simulink model "LdAfsSlave_Runner"  (R2020b)
settings: configuration reference "VLS_Standard_Configuration" (kept outside this file)
undefined symbols (not defined in the file): C_AfsRampTimeMatrix, C_CieCurveGammaToPwmY, C_CieCurvePwmToGammaY, C_DblSlavePeriod, C_EndIndexOfEachLightingModule, C_LedCenterDist, C_LedLeftDist, C_LedRightDist, C_StartIndexOfEachLightingModule
libraries: AfsSlaveLib x1
settings Model: DataDictionary=LdAfsDblSlaveDD.sldd  Creator=ahashem  LastModifiedBy=ahashem
settings ConfigSetRef: SourceName=VLS_Standard_Configuration

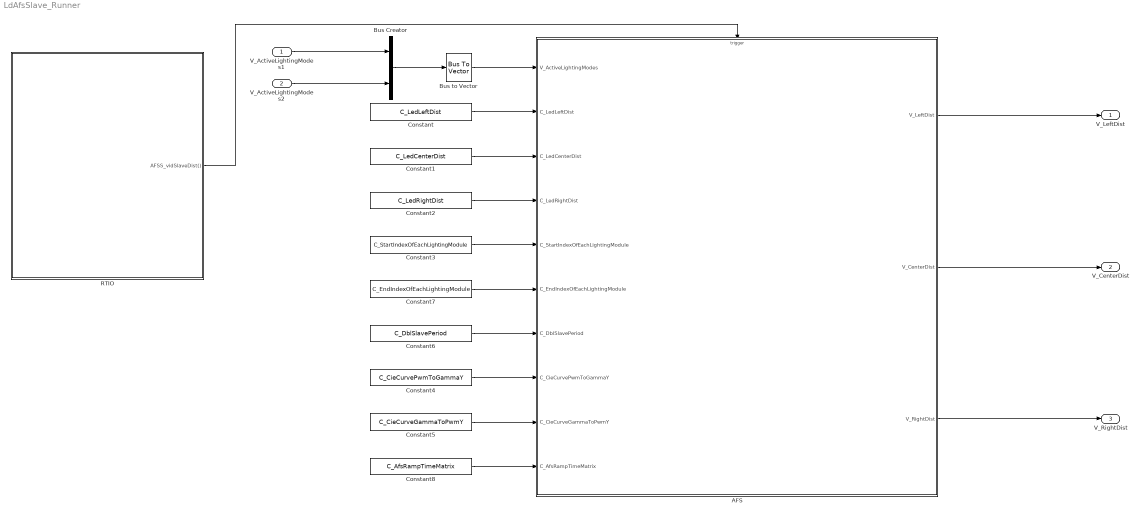
== system LdAfsSlave_Runner ==
  V_ActiveLightingModes1 : Inport
  V_ActiveLightingModes2 : Inport  Port=2
  AFS : Subsystem  Description=Clustering subsystem
  Bus Creator : BusCreator  Inputs=2
  Bus to Vector : BusToVector
  Constant : Constant  Value=C_LedLeftDist
  Constant1 : Constant  Value=C_LedCenterDist
  Constant2 : Constant  Value=C_LedRightDist
  Constant3 : Constant  Value=C_StartIndexOfEachLightingModule
  Constant4 : Constant  Value=C_CieCurvePwmToGammaY
  Constant5 : Constant  Value=C_CieCurveGammaToPwmY
  Constant6 : Constant  Value=C_DblSlavePeriod
  Constant7 : Constant  Value=C_EndIndexOfEachLightingModule
  Constant8 : Constant  Value=C_AfsRampTimeMatrix
  RTIO : Stateflow chart  TreatAsAtomicUnit=on  SystemSampleTime=0.02
  V_LeftDist : Outport  VectorParamsAs1DForOutWhenUnconnected=off
  V_CenterDist : Outport  Port=2  VectorParamsAs1DForOutWhenUnconnected=off
  V_RightDist : Outport  Port=3  VectorParamsAs1DForOutWhenUnconnected=off
  wires:
  Constant8/1 -> AFS/10(C_AfsRampTimeMatrix)
  Constant6/1 -> AFS/7(C_DblSlavePeriod)
  Constant5/1 -> AFS/9(C_CieCurveGammaToPwmY)
  Constant4/1 -> AFS/8(C_CieCurvePwmToGammaY)
  RTIO/1(AFSS_vidSlaveDist()) -> AFS/Trigger
  Constant2/1 -> AFS/4(C_LedRightDist)
  AFS/3(V_RightDist) -> V_RightDist/1
  AFS/2(V_CenterDist) -> V_CenterDist/1
  Bus Creator/1 -> Bus to Vector/1
  Constant3/1 -> AFS/5(C_StartIndexOfEachLightingModule)
  Constant1/1 -> AFS/3(C_LedCenterDist)
  AFS/1(V_LeftDist) -> V_LeftDist/1
  Constant7/1 -> AFS/6(C_EndIndexOfEachLightingModule)
  Constant/1 -> AFS/2(C_LedLeftDist)
  V_ActiveLightingModes2/1 -> Bus Creator/2
  V_ActiveLightingModes1/1 -> Bus Creator/1
  Bus to Vector/1 -> AFS/1(V_ActiveLightingModes)

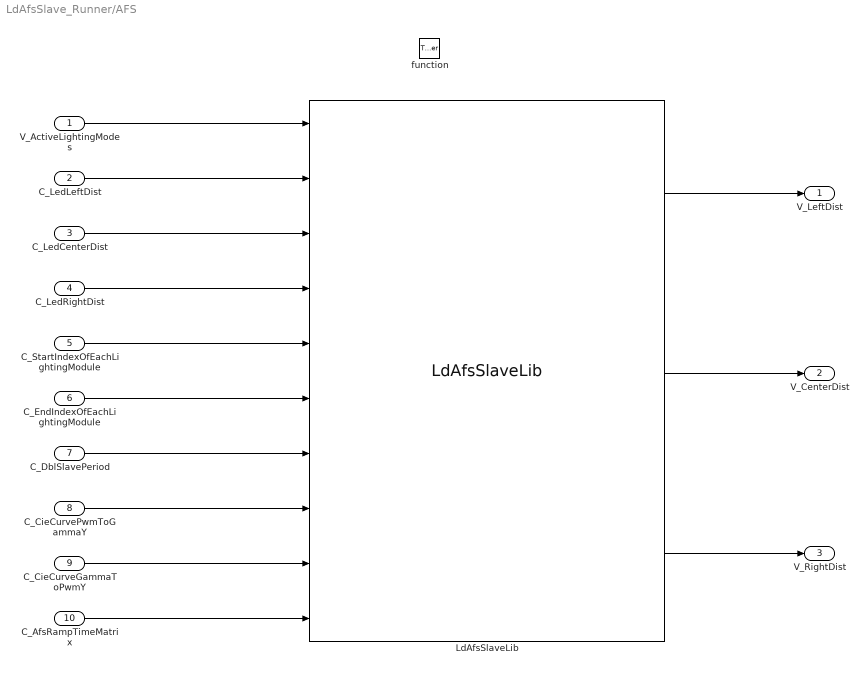
== system LdAfsSlave_Runner/AFS ==
  V_ActiveLightingModes : Inport
  C_LedLeftDist : Inport  Port=2
  C_LedCenterDist : Inport  Port=3
  C_LedRightDist : Inport  Port=4
  C_StartIndexOfEachLightingModule : Inport  Port=5
  C_EndIndexOfEachLightingModule : Inport  Port=6
  C_DblSlavePeriod : Inport  Port=7
  C_CieCurvePwmToGammaY : Inport  Port=8
  C_CieCurveGammaToPwmY : Inport  Port=9
  C_AfsRampTimeMatrix : Inport  Port=10
  function : TriggerPort  TriggerType=function-call  VariantControl=Variant
      settings: AttributesFormatString=StatesWhenEnabling: %<StatesWhenEnabling>
  LdAfsSlaveLib : AfsSlaveLib/LdAfsSlaveLib  SystemSampleTime=-1  VariantActivationTime=update diagram  Latency=0  AutoFrameSizeCalculation=off
  V_LeftDist : Outport  VectorParamsAs1DForOutWhenUnconnected=off
  V_CenterDist : Outport  Port=2  VectorParamsAs1DForOutWhenUnconnected=off
  V_RightDist : Outport  Port=3  VectorParamsAs1DForOutWhenUnconnected=off
  wires:
  V_ActiveLightingModes/1 -> LdAfsSlaveLib/1
  C_StartIndexOfEachLightingModule/1 -> LdAfsSlaveLib/5
  C_LedLeftDist/1 -> LdAfsSlaveLib/2
  C_LedCenterDist/1 -> LdAfsSlaveLib/3
  C_LedRightDist/1 -> LdAfsSlaveLib/4
  C_EndIndexOfEachLightingModule/1 -> LdAfsSlaveLib/6
  C_DblSlavePeriod/1 -> LdAfsSlaveLib/7
  C_CieCurvePwmToGammaY/1 -> LdAfsSlaveLib/8
  C_CieCurveGammaToPwmY/1 -> LdAfsSlaveLib/9
  C_AfsRampTimeMatrix/1 -> LdAfsSlaveLib/10
  LdAfsSlaveLib/3 -> V_RightDist/1
  LdAfsSlaveLib/2 -> V_CenterDist/1
  LdAfsSlaveLib/1 -> V_LeftDist/1

== stateflow chart LdAfsSlave_Runner/RTIO ==
  state Schedule
    on every(1,tick):
    send(AFSS_vidSlaveDist);
  (default) -> Schedule
  events: AFSS_vidSlaveDist output FUNCTION_CALL_EVENT
